simulink model "LCA_feature_mode"  (R2021a)
settings: Solver=VariableStepAuto  StartTime=0.0  StopTime=sim_time  RelTol=1e-3
values from neighbouring files (symbols this model uses):
  c_f = 155494.663    [LCA_init.m]    (also in MPC_init.m; week6_init.m)
  c_r = 1554494.663    [LCA_init.m]    (also in MPC_init.m; week6_init.m)
  I_z = 1436.24    [LCA_init.m]    (also in MPC_init.m; week6_init.m)
  L = 4.7    [LCA_init.m]    (also in LCA_lateral_movie_fcn.m = 5.7; PurePursuitModelInitialization.m; Pure_Pursiut_init.m; Stanley_control_init.m)
  l_f = 1.165    [LCA_init.m]    (also in MPC_init.m; week6_init.m)
  l_r = 1.165    [LCA_init.m]    (also in MPC_init.m; week6_init.m)
  ld = 15    [LCA_init.m]
  m = 1084    [Headway_Controller_Design.m]    (also in LCA_init.m = 1140; MPC_init.m = 1140; PID_Controller.m = 1; Reduced_order_model.m)
  md = get_curvature(Vx, yaw_rate_pose, tRef)    [LCA_init.m]
  Ts = 0.1    [LCA_init.m]    (also in MPC_init.m = 26; PurePursuitModelInitialization.m = 9; Pure_Pursiut_init.m = 9; Stanley_control_init.m = 1.6)
  Vx = 25    [LCA_init.m]    (also in MPC_init.m = 10; week6_init.m = 30)
  xRef = refPose(1,:)    [LCA_init.m]    (also in MPC_init.m; PurePursuitModelInitialization.m = refPose(:,1); Pure_Pursiut_init.m; Stanley_control_init.m = refpose(1,:))
  yRef = refPose(2,:) + 2    [LCA_init.m]    (also in MPC_init.m; PurePursuitModelInitialization.m = -refPose(:,2); Pure_Pursiut_init.m = refPose(2,:); Stanley_control_init.m = refpose(2,:))
undefined symbols (not defined in the file or in its folder): sigbuilder_block
libraries: simulink x2, mpcadaslib x1, robotalgslib x1, autolibshared x1
settings Model: Creator=User  LastModifiedBy=User

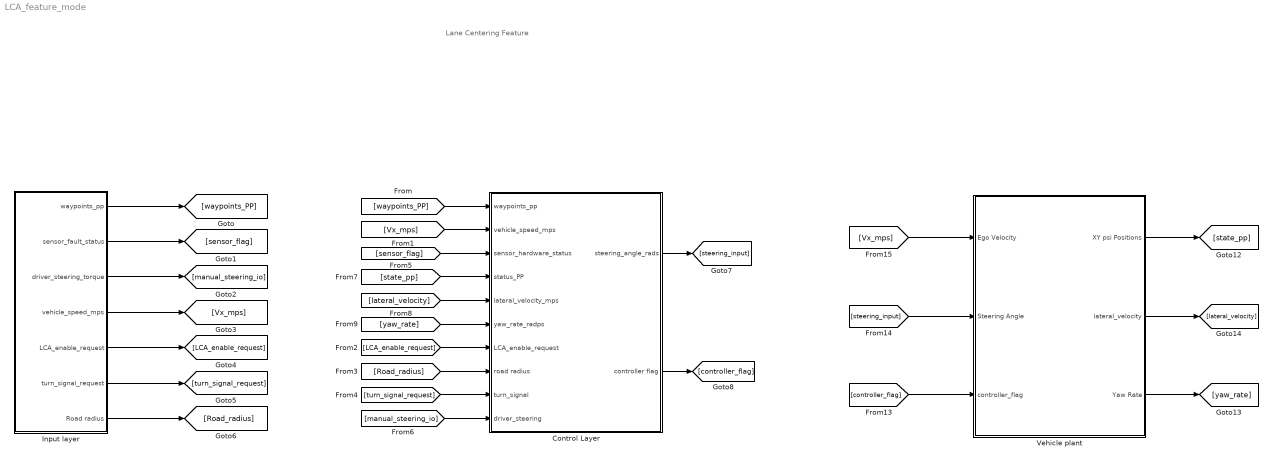
== system LCA_feature_mode ==
  note: Lane Centering Feature
  "\tControl Layer" : Subsystem
  Input layer : Subsystem
  Vehicle plant : Subsystem
  wires:
  Input layer/1(waypoints_pp) -> [waypoints_PP]
  Input layer/2(sensor_fault_status) -> [sensor_flag]
  Input layer/3(driver_steering_torque) -> [manual_steering_io]
  Input layer/4(vehicle_speed_mps) -> [Vx_mps]
  Input layer/5(LCA_enable_request) -> [LCA_enable_request]
  Input layer/6(turn_signal_request) -> [turn_signal_request]
  Input layer/7(Road radius) -> [Road_radius]
  [waypoints_PP] -> "\tControl Layer"/1(waypoints_pp)
  [Vx_mps] -> "\tControl Layer"/2(vehicle_speed_mps)
  [LCA_enable_request] -> "\tControl Layer"/7(LCA_enable_request)
  [Road_radius] -> "\tControl Layer"/8(road radius)
  [turn_signal_request] -> "\tControl Layer"/9(turn_signal)
  [sensor_flag] -> "\tControl Layer"/3(sensor_hardware_status)
  [manual_steering_io] -> "\tControl Layer"/10(driver_steering)
  [state_pp] -> "\tControl Layer"/4(status_PP)
  [lateral_velocity] -> "\tControl Layer"/5(lateral_velocity_mps)
  [yaw_rate] -> "\tControl Layer"/6(yaw_rate_radps)
  "\tControl Layer"/1(steering_angle_rads) -> [steering_input]
  "\tControl Layer"/2(controller flag) -> [controller_flag]
  Vehicle plant/1(XY psi Positions) -> [state_pp]
  Vehicle plant/3(Yaw Rate) -> [yaw_rate]
  [steering_input] -> Vehicle plant/2(Steering Angle)
  [Vx_mps] -> Vehicle plant/1(Ego Velocity)
  Vehicle plant/2(lateral_velocity) -> [lateral_velocity]
  [controller_flag] -> Vehicle plant/3(controller_flag)

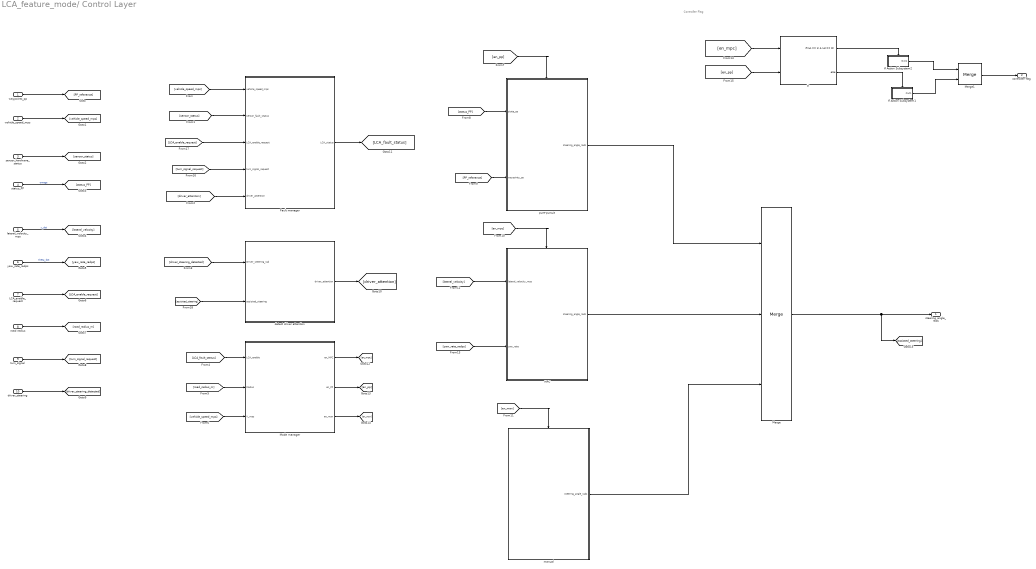
== system LCA_feature_mode/	Control Layer ==
  note: Controller Flag
  waypoints_pp : Inport
  vehicle_speed_mps : Inport  Port=2
  sensor_hardware_status : Inport  Port=3
  status_PP : Inport  Port=4
  lateral_velocity_mps : Inport  Port=5
  yaw_rate_radps : Inport  Port=6
  LCA_enable_request : Inport  Port=7
  road radius : Inport  Port=8
  turn_signal : Inport  Port=9
  driver_steering : Inport  Port=10
  Fault manager : Subsystem
  If : If  NumInputs=2  IfExpression=(u1 == 1) & (u2 == 0)
  If Action Subsystem1 : Subsystem  TreatAsAtomicUnit=on
  If Action Subsystem2 : Subsystem  TreatAsAtomicUnit=on
  MPC : Subsystem
  Merge : Merge  Inputs=3
  Merge1 : Merge
  Mode manager : Subsystem
  detect driver attention : Subsystem
  manual : Subsystem
  pure-pursuit : Subsystem
  steering_angle_rads : Outport
  controller flag : Outport  Port=2
  wires:
  waypoints_pp/1 -> [PP_reference]
  vehicle_speed_mps/1 -> [vehicle_speed_mps]
  sensor_hardware_status/1 -> [sensor_status]
  status_PP/1 -> [status_PP]  "omega"
  lateral_velocity_mps/1 -> [lateral_velocity]  "y_dot"
  yaw_rate_radps/1 -> [yaw_rate_radps]  "theta_dot"
  LCA_enable_request/1 -> [LCA_enable_request]
  road radius/1 -> [road_radius_m]
  turn_signal/1 -> [turn_signal_request]
  driver_steering/1 -> [driver_steering_detected]
  [vehicle_speed_mps] -> Fault manager/1(vehicle_speed_mps)
  [sensor_status] -> Fault manager/2(sensor_fault_status)
  detect driver attention/1(driver_attention) -> [driver_attention]
  [driver_attention] -> Fault manager/5("\tdriver_attention")
  [driver_steering_detected] -> detect driver attention/1(Driver_steering_rad)
  Fault manager/1(LCA_status) -> [LCA_fault_status]
  [LCA_fault_status] -> Mode manager/1(LCA_enable)
  [road_radius_m] -> Mode manager/2(Radius)
  [vehicle_speed_mps] -> Mode manager/3(V_mps)
  Mode manager/1(en_MPC) -> [en_mpc]
  Mode manager/2(en_PP) -> [en_pp]
  Mode manager/3(en_man) -> [en_man]
  [en_pp] -> pure-pursuit/Enable
  [status_PP] -> pure-pursuit/1(state_pp)
  [PP_reference] -> pure-pursuit/2(waypoints_pp)
  pure-pursuit/1(steering_angle_rads) -> Merge/1
  MPC/1(steering_angle_rads) -> Merge/2
  [en_mpc] -> MPC/Enable
  [en_man] -> manual/Enable
  manual/1(steering_angle_rads) -> Merge/3
  Merge/1 -> [assisted_steering], steering_angle_rads/1
  [lateral_velocity] -> MPC/1(lateral_velocity_mps)
  [yaw_rate_radps] -> MPC/2(yaw_rate)
  [en_mpc] -> If/1
  [en_pp] -> If/2
  If/1 -> If Action Subsystem2/Action
  If Action Subsystem2/1(Out1) -> Merge1/1
  Merge1/1 -> controller flag/1
  If/2 -> If Action Subsystem1/Action
  If Action Subsystem1/1(Out1) -> Merge1/2
  [turn_signal_request] -> Fault manager/4("\tturn_signal_request")
  [LCA_enable_request] -> Fault manager/3("\tLCA_enable_request")
  [assisted_steering] -> detect driver attention/2(assisted_steering)

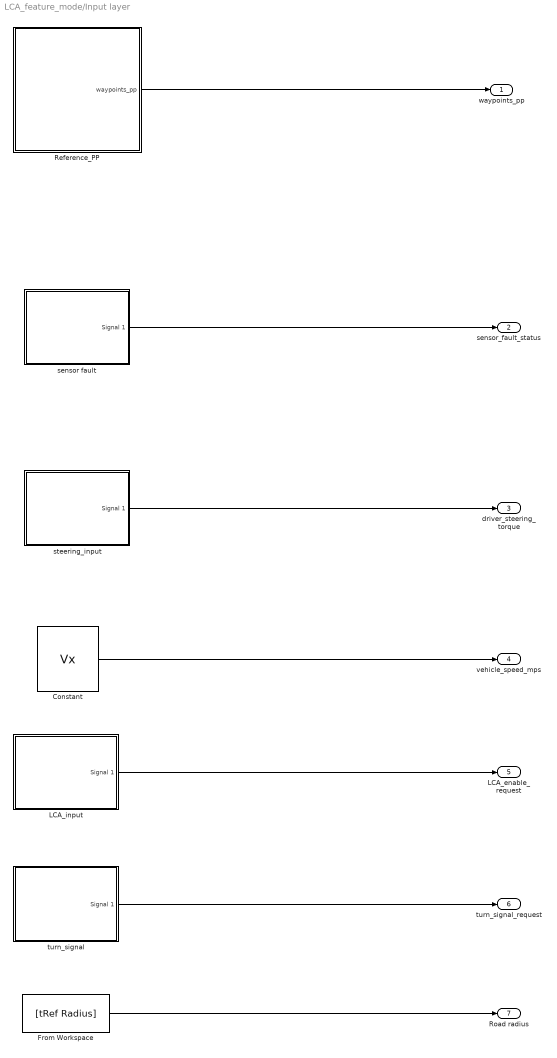
== system LCA_feature_mode/Input layer ==
  Constant : Constant  Value=Vx
  From Workspace : FromWorkspace  VariableName=[tRef Radius]  SampleTime=0.1
  LCA_input : Subsystem  Tag=STV Subsys  LoadFcn=sigbuilder_block('load');  StartFcn=sigbuilder_block('start');  StopFcn=sigbuilder_block('stop');  ClipboardFcn=sigbuilder_block('clipboard');  mask(Sigbuilder block){tuvar=[0:10]}
      mask help: Simulink:masks:SigbuilderBlock_MD
      mask init:
      | if ~strcmp(get_param(bdroot(gcbh),'SimulationStatus'),'stopped') tuvar = sigbuilder_block('maskInit'); end
      settings: CopyFcn=sigbuilder_block('copy');  DeleteFcn=sigbuilder_block('delete');  ModelCloseFcn=sigbuilder_block('modelClose');  PreSaveFcn=sigbuilder_block('preSave');  PauseFcn=sigbuilder_block('pause');  ContinueFcn=sigbuilder_block('continue');  NameChangeFcn=sigbuilder_block('namechange');  OpenFcn=sigbuilder_block('open',[309 216.75 550.5 359.25 ]);  CloseFcn=sigbuilder_block('close');
      mask Display: plot(0, 0, 100, 100,[2, 2, 32, 32, 2], [68, 8, 8, 68, 68],[32, 2], [38, 38], [32, 19, 2],[53, 60, 44], [32, 17, 17, 2],[16, 16, 31, 31]);txt = getActiveGroup(gcbh);text(2, 100, txt,'verticalAlignment', 'top');
  Reference_PP : Subsystem
  sensor fault : Subsystem  Tag=STV Subsys  LoadFcn=sigbuilder_block('load');  StartFcn=sigbuilder_block('start');  StopFcn=sigbuilder_block('stop');  ClipboardFcn=sigbuilder_block('clipboard');  mask(Sigbuilder block){tuvar=[0:10]}
      mask help: Simulink:masks:SigbuilderBlock_MD
      mask init:
      | if ~strcmp(get_param(bdroot(gcbh),'SimulationStatus'),'stopped') tuvar = sigbuilder_block('maskInit'); end
      settings: CopyFcn=sigbuilder_block('copy');  DeleteFcn=sigbuilder_block('delete');  ModelCloseFcn=sigbuilder_block('modelClose');  PreSaveFcn=sigbuilder_block('preSave');  PauseFcn=sigbuilder_block('pause');  ContinueFcn=sigbuilder_block('continue');  NameChangeFcn=sigbuilder_block('namechange');  OpenFcn=sigbuilder_block('open',[309 216.75 550.5 359.25 ]);  CloseFcn=sigbuilder_block('close');
      mask Display: plot(0, 0, 100, 100,[2, 2, 32, 32, 2], [68, 8, 8, 68, 68],[32, 2], [38, 38], [32, 19, 2],[53, 60, 44], [32, 17, 17, 2],[16, 16, 31, 31]);txt = getActiveGroup(gcbh);text(2, 100, txt,'verticalAlignment', 'top');
  steering_input : Subsystem  Tag=STV Subsys  LoadFcn=sigbuilder_block('load');  StartFcn=sigbuilder_block('start');  StopFcn=sigbuilder_block('stop');  ClipboardFcn=sigbuilder_block('clipboard');  mask(Sigbuilder block){tuvar=[0:10]}
      mask help: Simulink:masks:SigbuilderBlock_MD
      mask init:
      | if ~strcmp(get_param(bdroot(gcbh),'SimulationStatus'),'stopped') tuvar = sigbuilder_block('maskInit'); end
      settings: CopyFcn=sigbuilder_block('copy');  DeleteFcn=sigbuilder_block('delete');  ModelCloseFcn=sigbuilder_block('modelClose');  PreSaveFcn=sigbuilder_block('preSave');  PauseFcn=sigbuilder_block('pause');  ContinueFcn=sigbuilder_block('continue');  NameChangeFcn=sigbuilder_block('namechange');  OpenFcn=sigbuilder_block('open',[309 216.75 550.5 359.25 ]);  CloseFcn=sigbuilder_block('close');
      mask Display: plot(0, 0, 100, 100,[2, 2, 32, 32, 2], [68, 8, 8, 68, 68],[32, 2], [38, 38], [32, 19, 2],[53, 60, 44], [32, 17, 17, 2],[16, 16, 31, 31]);txt = getActiveGroup(gcbh);text(2, 100, txt,'verticalAlignment', 'top');
  turn_signal : Subsystem  Tag=STV Subsys  LoadFcn=sigbuilder_block('load');  StartFcn=sigbuilder_block('start');  StopFcn=sigbuilder_block('stop');  ClipboardFcn=sigbuilder_block('clipboard');  mask(Sigbuilder block){tuvar=[0:10]}
      mask help: Simulink:masks:SigbuilderBlock_MD
      mask init:
      | if ~strcmp(get_param(bdroot(gcbh),'SimulationStatus'),'stopped') tuvar = sigbuilder_block('maskInit'); end
      settings: CopyFcn=sigbuilder_block('copy');  DeleteFcn=sigbuilder_block('delete');  ModelCloseFcn=sigbuilder_block('modelClose');  PreSaveFcn=sigbuilder_block('preSave');  PauseFcn=sigbuilder_block('pause');  ContinueFcn=sigbuilder_block('continue');  NameChangeFcn=sigbuilder_block('namechange');  OpenFcn=sigbuilder_block('open',[309 216.75 550.5 359.25 ]);  CloseFcn=sigbuilder_block('close');
      mask Display: plot(0, 0, 100, 100,[2, 2, 32, 32, 2], [68, 8, 8, 68, 68],[32, 2], [38, 38], [32, 19, 2],[53, 60, 44], [32, 17, 17, 2],[16, 16, 31, 31]);txt = getActiveGroup(gcbh);text(2, 100, txt,'verticalAlignment', 'top');
  waypoints_pp : Outport
  sensor_fault_status : Outport  Port=2
  driver_steering_torque : Outport  Port=3
  vehicle_speed_mps : Outport  Port=4
  LCA_enable_request : Outport  Port=5
  turn_signal_request : Outport  Port=6
  Road radius : Outport  Port=7
  wires:
  Reference_PP/1(waypoints_pp) -> waypoints_pp/1
  sensor fault/1(Signal 1) -> sensor_fault_status/1
  steering_input/1(Signal 1) -> driver_steering_torque/1
  Constant/1 -> vehicle_speed_mps/1
  LCA_input/1(Signal 1) -> LCA_enable_request/1
  turn_signal/1(Signal 1) -> turn_signal_request/1
  From Workspace/1 -> Road radius/1

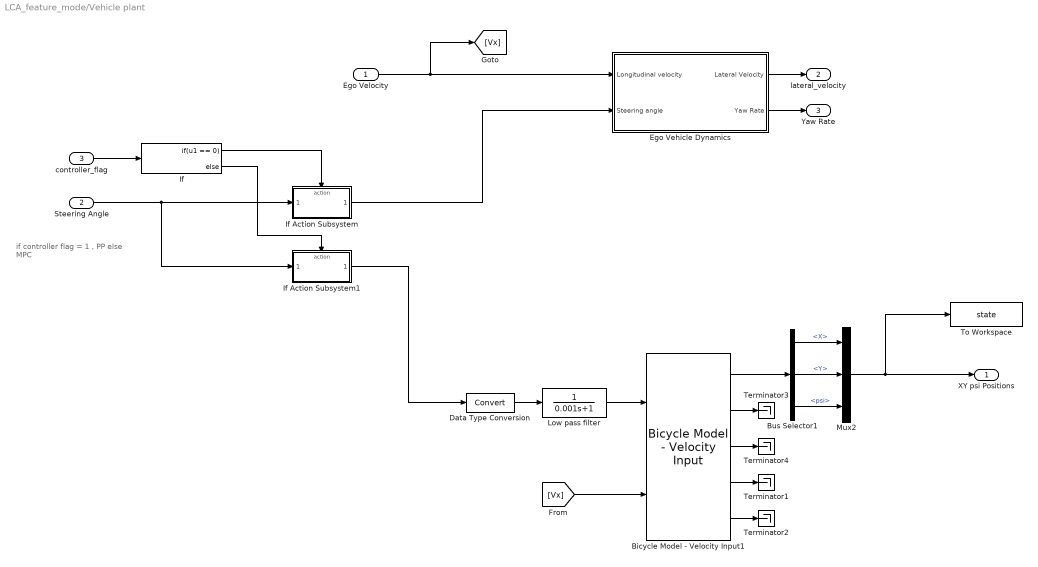
== system LCA_feature_mode/Vehicle plant ==
  note: if controller flag = 1 , PP
      | else MPC
  Ego Velocity : Inport
  Steering Angle : Inport  Port=2
  controller_flag : Inport  Port=3
  Bicycle Model - Velocity Input1 : autolibshared/Bicycle Model - Velocity Input  trackMode=Single (bicycle)  inputMode=External longitudinal forces  frontSteerMode=on  rearSteerMode=off  windMode=off  muMode=off  extFMode=off  extMMode=off  aMode=3  NF=2  NR=2  m=m  a=l_f  b=l_r  h=0.35  X_o=X_o  xdot_o=0  CalphaMode=off  sigmaMode=on  w=[1.4,1.4]  Cy_f=c_f  Cy_r=c_r  sigma_f=.1  sigma_r=.1  alpha_f_brk=[-.1 .1]  Cy_f_data=[-9e3 9e3]  alpha_r_brk=[-.1 .1]  Cy_r_data=[-9e3 9e3]  Y_o=Y_o  ydot_o=0  Izz=I_z  psi_o=0  r_o=0  Af=2  Cd=.3  Cl=.1  Cpm=.1  beta_w=[0:0.01:0.3]  Cs=[0:0.03:0.9]  Cym=[0:0.01:0.3]  Pabs=101325  Tair=273  g=9.81  mu=1  xdot_tol=.01  Fznom=5000  Fxtire_sat=1e6  Fytire_sat=1e6  longOff=0  latOff=0  vertOff=0
      settings: SourceProductBaseCode=PW,MT,UV,VE,VP
  Bus Selector1 : BusSelector  OutputSignals=InertFrm.FrntAxl.Disp.X,InertFrm.FrntAxl.Disp.Y,InertFrm.Cg.Ang.psi
  Data Type Conversion : DataTypeConversion
  Ego Vehicle Dynamics : Subsystem
  If : If  IfExpression=u1 == 0
  If Action Subsystem : Subsystem  TreatAsAtomicUnit=on
  If Action Subsystem1 : Subsystem  TreatAsAtomicUnit=on
  Low pass filter : TransferFcn  Denominator=[0.001 1]
  Mux2 : Mux  Inputs=3
  Terminator{1..4} (4 alike) : Terminator
  To Workspace : ToWorkspace  VariableName=state  SampleTime=-1
  XY psi Positions : Outport  Unit=m  VectorParamsAs1DForOutWhenUnconnected=off
  lateral_velocity : Outport  Port=2  Unit=m/s  VectorParamsAs1DForOutWhenUnconnected=off
  Yaw Rate : Outport  Port=3  Unit=degree/s  VectorParamsAs1DForOutWhenUnconnected=off
  wires:
  Bicycle Model - Velocity Input1/3 -> Terminator4/1
  Bicycle Model - Velocity Input1/2 -> Terminator3/1
  Data Type Conversion/1 -> Low pass filter/1
  Mux2/1 -> To Workspace/1, XY psi Positions/1
  Bicycle Model - Velocity Input1/1 -> Bus Selector1/1
  Low pass filter/1 -> Bicycle Model - Velocity Input1/1
  Bicycle Model - Velocity Input1/5 -> Terminator2/1
  Bus Selector1/1 -> Mux2/1  "<X>"
  Bus Selector1/2 -> Mux2/2  "<Y>"
  Bicycle Model - Velocity Input1/4 -> Terminator1/1
  Bus Selector1/3 -> Mux2/3  "<psi>"
  Ego Velocity/1 -> [Vx], Ego Vehicle Dynamics/1(Longitudinal velocity)
  Ego Vehicle Dynamics/2(Yaw Rate) -> Yaw Rate/1
  Ego Vehicle Dynamics/1(Lateral Velocity) -> lateral_velocity/1
  [Vx] -> Bicycle Model - Velocity Input1/2
  controller_flag/1 -> If/1
  Steering Angle/1 -> If Action Subsystem1/1(Steering Angle), If Action Subsystem/1(Steering Angle)
  If/1 -> If Action Subsystem/Action
  If/2 -> If Action Subsystem1/Action
  If Action Subsystem/1(steering angle to ego dynamics) -> Ego Vehicle Dynamics/2(Steering angle)
  If Action Subsystem1/1(wheenangle) -> Data Type Conversion/1

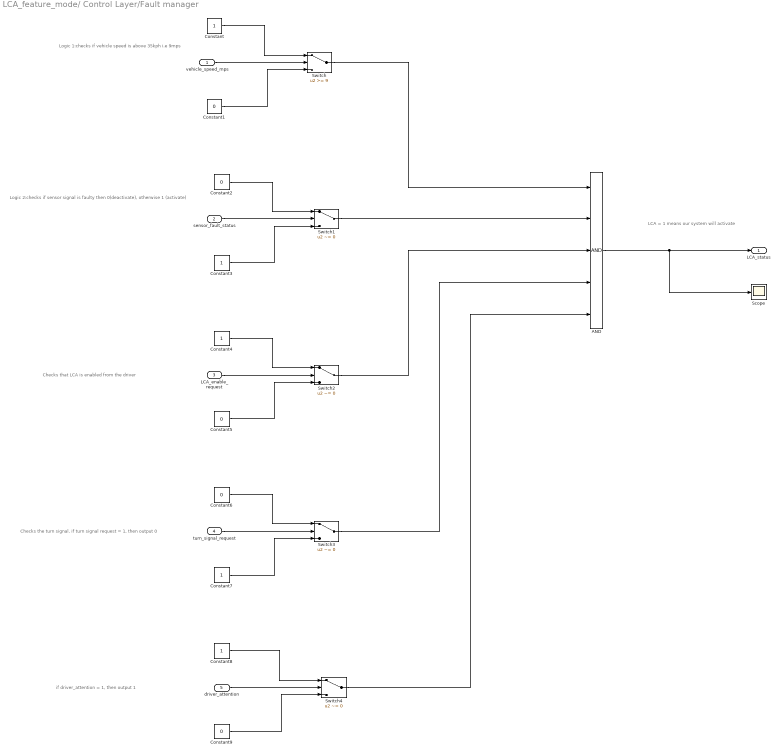
== system LCA_feature_mode/	Control Layer/Fault manager ==
  note: Logic 1:checks if vehicle speed is above 35kph i.e 9mps
  note: Logic 2:checks if sensor signal is faulty then 0(deactivate), otherwise 1 (activate)
  note: Checks that LCA is enabled from the driver
  note: Checks the turn signal. if turn signal request = 1, then output 0
  note: if driver_attention = 1, then output 1
  note: LCA = 1 means our system will activate
  vehicle_speed_mps : Inport
  sensor_fault_status : Inport  Port=2
  "\tLCA_enable_request" : Inport  Port=3
  "\tturn_signal_request" : Inport  Port=4
  "\tdriver_attention" : Inport  Port=5
  AND : Logic  Inputs=5  AllPortsSameDT=off  OutDataTypeStr=boolean
  Constant{,3..4,7..8} (5 alike) : Constant
  Constant{1..2,5..6,9} (5 alike) : Constant  Value=0
  Scope : Scope
  Switch : Switch  Threshold=9
  Switch{1..4} (4 alike) : Switch  Criteria=u2 ~= 0
  LCA_status : Outport
  wires:
  vehicle_speed_mps/1 -> Switch/2
  Constant/1 -> Switch/1
  Constant1/1 -> Switch/3
  Constant3/1 -> Switch1/3
  Constant2/1 -> Switch1/1
  sensor_fault_status/1 -> Switch1/2
  "\tLCA_enable_request"/1 -> Switch2/2
  Constant4/1 -> Switch2/1
  Constant5/1 -> Switch2/3
  Constant7/1 -> Switch3/3
  Constant6/1 -> Switch3/1
  "\tturn_signal_request"/1 -> Switch3/2
  "\tdriver_attention"/1 -> Switch4/2
  Constant8/1 -> Switch4/1
  Constant9/1 -> Switch4/3
  Switch/1 -> AND/1
  Switch1/1 -> AND/2
  Switch2/1 -> AND/3
  Switch3/1 -> AND/4
  Switch4/1 -> AND/5
  AND/1 -> Scope/1, LCA_status/1

== system LCA_feature_mode/	Control Layer/If Action Subsystem1 ==
  Action Port : ActionPort  ActionPortLabel=else
  Constant : Constant
  Out1 : Outport
  wires:
  Constant/1 -> Out1/1

== system LCA_feature_mode/	Control Layer/If Action Subsystem2 ==
  Action Port : ActionPort  ActionPortLabel=if((u1 == 1) & (u2 == 0))
  Constant : Constant
  Out1 : Outport
  wires:
  Constant/1 -> Out1/1

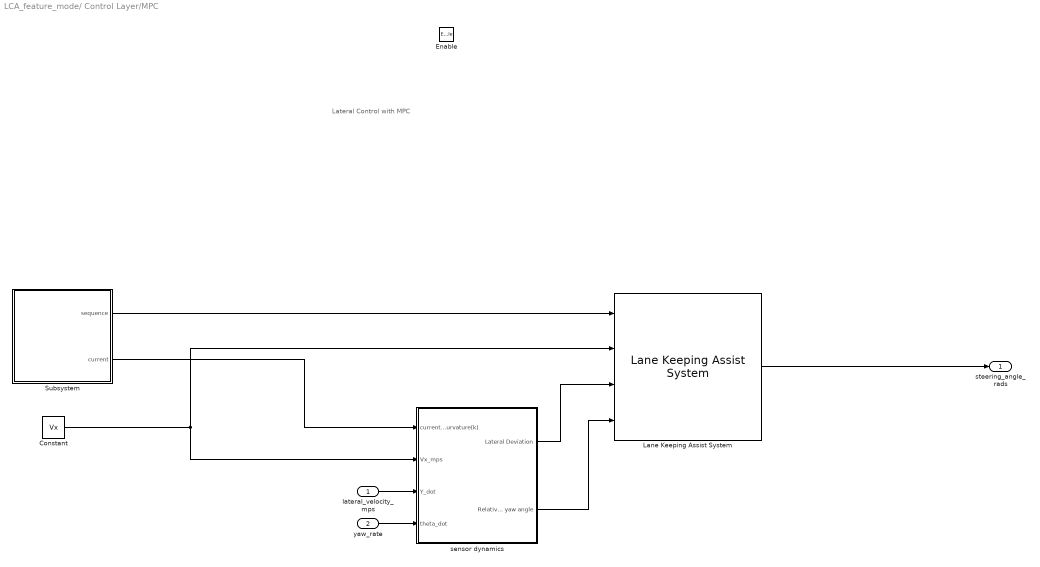
== system LCA_feature_mode/	Control Layer/MPC ==
  note: Lateral Control with MPC
  lateral_velocity_mps : Inport
  yaw_rate : Inport  Port=2
  Enable : EnablePort
  Constant : Constant  Value=Vx
  Lane Keeping Assist System : mpcadaslib/Lane Keeping Assist System  ModelType=Use vehicle parameters  VehicleMass=m  VehicleYawInertia=I_z  LengthToFront=l_f  LengthToRear=l_r  FrontTireStiffness=c_f  RearTireStiffness=c_r  EgoModelMatrixA=[-4.4021 ,-12.4603;1.3913,-5.1868]  EgoModelMatrixB=[24.1270;15.8609]  EgoModelMatrixC=[1,0;0,1]  InitialLongVel=Vx  TransportLag=0  MinSteering=-0.5  umin_ext=off  MaxSteering=0.5  umax_ext=off  Ts=0.1  PredictionHorizon=10  ControllerBehavior=0.500  suboptimal=off  maxiter=10  datatypeopt=double  optmode=off  trackmode=off
      settings: SourceProductBaseCode=MP
  Subsystem : Subsystem  mask{signal=md, ts=Ts, steps=10}
      mask prompts: signal "Signal name"; ts "Sampling time"; steps "Number of previewing steps"
      mask init:
      | ts = evalin('base',get_param(gcbh,'ts'));
      | signal = evalin('base',get_param(gcbh,'signal'));
      | steps = evalin('base',get_param(gcbh,'steps'));
      | data = mpc_previewer_maskinit(signal,ts);
      mask Display:
      | fprintf('Future\nsample\nextractor');
      | port_label('output', 1, 'seq')
      | port_label('output', 2, '@t')
  sensor dynamics : Subsystem
  steering_angle_rads : Outport
  wires:
  Lane Keeping Assist System/1 -> steering_angle_rads/1
  Constant/1 -> sensor dynamics/2(Vx_mps), Lane Keeping Assist System/2
  sensor dynamics/1(Lateral Deviation) -> Lane Keeping Assist System/3
  sensor dynamics/2(Relative yaw angle) -> Lane Keeping Assist System/4
  lateral_velocity_mps/1 -> sensor dynamics/3(Y_dot)
  yaw_rate/1 -> sensor dynamics/4(theta_dot)
  Subsystem/2(current) -> sensor dynamics/1(current_curvature(k))
  Subsystem/1(sequence) -> Lane Keeping Assist System/1

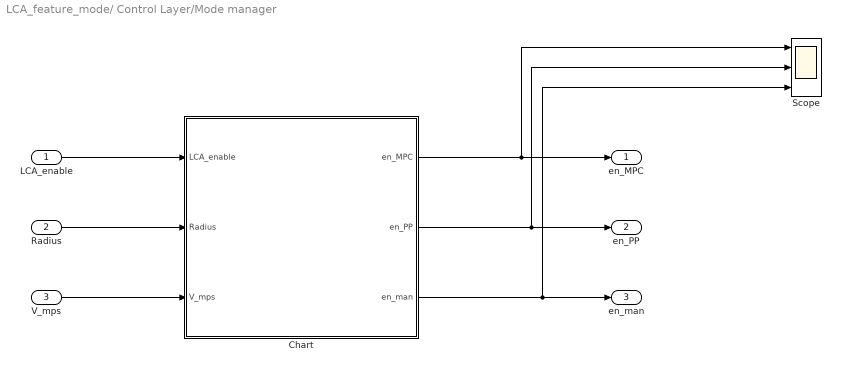
== system LCA_feature_mode/	Control Layer/Mode manager ==
  LCA_enable : Inport
  Radius : Inport  Port=2
  V_mps : Inport  Port=3
  Chart : Stateflow chart  TreatAsAtomicUnit=on
  Scope : Scope  NumInputPorts=3
  en_MPC : Outport
  en_PP : Outport  Port=2
  en_man : Outport  Port=3
  wires:
  LCA_enable/1 -> Chart/1(LCA_enable)
  Radius/1 -> Chart/2(Radius)
  V_mps/1 -> Chart/3(V_mps)
  Chart/1(en_MPC) -> Scope/1, en_MPC/1
  Chart/2(en_PP) -> Scope/2, en_PP/1
  Chart/3(en_man) -> Scope/3, en_man/1

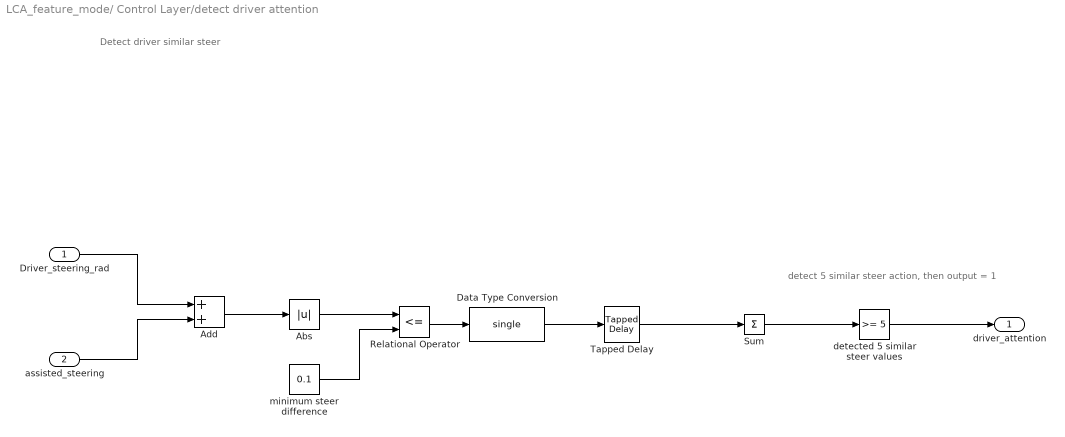
== system LCA_feature_mode/	Control Layer/detect driver attention ==
  note: detect 5 similar steer action, then output = 1
  note: Detect driver similar steer
  Driver_steering_rad : Inport
  assisted_steering : Inport  Port=2
  Abs : Abs
  Add : Sum
  Data Type Conversion : DataTypeConversion  OutDataTypeStr=single
  Relational Operator : RelationalOperator  Operator=<=  OutDataTypeStr=boolean  RndMeth=Simplest
  Sum : Sum  Inputs=+
  Tapped Delay : simulink/Discrete/Tapped Delay  vinit=0.0  samptime=-1  NumDelays=5  DelayOrder=Oldest  includeCurrent=off
  detected 5 similar steer values : simulink/Logic and Bit Operations/Compare To Constant  relop=>=  const=5  OutDataTypeStr=boolean
  minimum steer difference : Constant  Value=0.1
  driver_attention : Outport
  wires:
  Driver_steering_rad/1 -> Add/1
  assisted_steering/1 -> Add/2
  Add/1 -> Abs/1
  Abs/1 -> Relational Operator/1
  minimum steer difference/1 -> Relational Operator/2
  Relational Operator/1 -> Data Type Conversion/1
  Data Type Conversion/1 -> Tapped Delay/1
  Tapped Delay/1 -> Sum/1
  Sum/1 -> detected 5 similar steer values/1
  detected 5 similar steer values/1 -> driver_attention/1

== system LCA_feature_mode/	Control Layer/manual ==
  Enable : EnablePort
  Constant : Constant  Value=0
  steering_angle_rads : Outport
  wires:
  Constant/1 -> steering_angle_rads/1

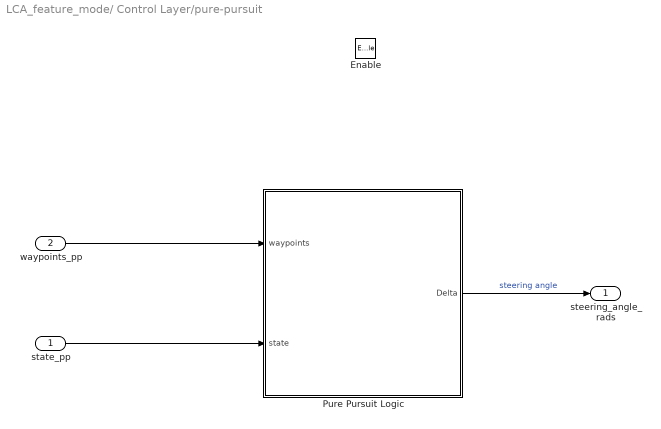
== system LCA_feature_mode/	Control Layer/pure-pursuit ==
  state_pp : Inport
  waypoints_pp : Inport  Port=2
  Enable : EnablePort
  Pure Pursuit Logic : Subsystem
  steering_angle_rads : Outport
  wires:
  state_pp/1 -> Pure Pursuit Logic/2(state)
  waypoints_pp/1 -> Pure Pursuit Logic/1(waypoints)
  Pure Pursuit Logic/1(Delta) -> steering_angle_rads/1  "steering angle"

== system LCA_feature_mode/Input layer/LCA_input ==
  Demux : Demux  Tag=STV Demux  Outputs=1
      settings: DisplayOption=none
  FromWs : FromWorkspace  Tag=STV FromWs  VariableName=tuvar
      SigBuilderData=|
      | common.afterFinalStr = 'Extrapolate'
      | common.sampleTime = 0
      | dataSet.timeRange = [0 10]
      | dataSet.name = 'Group 1'
      | sbobj.Groups.Name = 'Group 1'
      | sbobj.Groups.Signals.Name = 'Signal 1'
      | sbobj.Groups.Signals.XData = [0 4 4 6 6 10]
      | sbobj.Groups.Signals.YData = [0 0 1 1 0 0]
  Signal 1 : Outport  Tag=STV Outport
  wires:
  Demux/1 -> Signal 1/1
  FromWs/1 -> Demux/1

== system LCA_feature_mode/Input layer/Reference_PP ==
  Constant : Constant  Value=xRef  SampleTime=0.1
  Constant1 : Constant  Value=yRef  SampleTime=0.1
  Matrix Concatenate : Concatenate  Mode=Multidimensional array  ConcatenateDimension=2
  waypoints_pp : Outport
  wires:
  Constant/1 -> Matrix Concatenate/1
  Constant1/1 -> Matrix Concatenate/2
  Matrix Concatenate/1 -> waypoints_pp/1

== system LCA_feature_mode/Input layer/sensor fault ==
  Demux : Demux  Tag=STV Demux  Outputs=1
      settings: DisplayOption=none
  FromWs : FromWorkspace  Tag=STV FromWs  VariableName=tuvar
      SigBuilderData=|
      | common.afterFinalStr = 'Extrapolate'
      | common.sampleTime = 0
      | dataSet.timeRange = [0 10]
      | dataSet.name = 'Group 1'
      | sbobj.Groups.Name = 'Group 1'
      | sbobj.Groups.Signals.Name = 'Signal 1'
      | sbobj.Groups.Signals.XData = [0 4 4 6 6 10]
      | sbobj.Groups.Signals.YData = [0 0 1 1 0 0]
  Signal 1 : Outport  Tag=STV Outport
  wires:
  Demux/1 -> Signal 1/1
  FromWs/1 -> Demux/1

== system LCA_feature_mode/Input layer/steering_input ==
  Demux : Demux  Tag=STV Demux  Outputs=1
      settings: DisplayOption=none
  FromWs : FromWorkspace  Tag=STV FromWs  VariableName=tuvar
      SigBuilderData=|
      | common.afterFinalStr = 'Extrapolate'
      | common.sampleTime = 0
      | dataSet.timeRange = [0 10]
      | dataSet.name = 'Group 1'
      | sbobj.Groups.Name = 'Group 1'
      | sbobj.Groups.Signals.Name = 'Signal 1'
      | sbobj.Groups.Signals.XData = [0 4 4 6 6 10]
      | sbobj.Groups.Signals.YData = [0 0 1 1 0 0]
  Signal 1 : Outport  Tag=STV Outport
  wires:
  FromWs/1 -> Demux/1
  Demux/1 -> Signal 1/1

== system LCA_feature_mode/Input layer/turn_signal ==
  Demux : Demux  Tag=STV Demux  Outputs=1
      settings: DisplayOption=none
  FromWs : FromWorkspace  Tag=STV FromWs  VariableName=tuvar
      SigBuilderData=|
      | common.afterFinalStr = 'Extrapolate'
      | common.sampleTime = 0
      | dataSet.timeRange = [0 10]
      | dataSet.name = 'Group 1'
      | sbobj.Groups.Name = 'Group 1'
      | sbobj.Groups.Signals.Name = 'Signal 1'
      | sbobj.Groups.Signals.XData = [0 4 4 6 6 10]
      | sbobj.Groups.Signals.YData = [0 0 1 1 0 0]
  Signal 1 : Outport  Tag=STV Outport
  wires:
  FromWs/1 -> Demux/1
  Demux/1 -> Signal 1/1

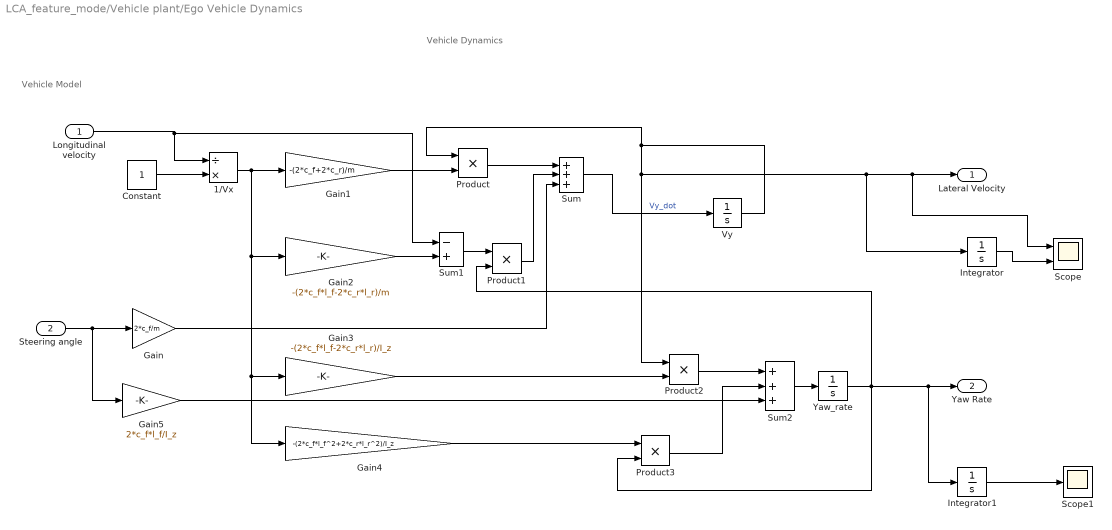
== system LCA_feature_mode/Vehicle plant/Ego Vehicle Dynamics ==
  note: Vehicle Model
  note: Vehicle Dynamics
  Longitudinal velocity : Inport
  Steering angle : Inport  Port=2
  1/Vx : Product  Inputs=/*
  Constant : Constant
  Gain : Gain  Gain=2*c_f/m
  Gain1 : Gain  Gain=-(2*c_f+2*c_r)/m
  Gain2 : Gain  Gain=-(2*c_f*l_f-2*c_r*l_r)/m
  Gain3 : Gain  Gain=-(2*c_f*l_f-2*c_r*l_r)/I_z
  Gain4 : Gain  Gain=-(2*c_f*l_f^2+2*c_r*l_r^2)/I_z
  Gain5 : Gain  Gain=2*c_f*l_f/I_z
  Integrator : Integrator
  Integrator1 : Integrator
  Product{,1..3} (4 alike) : Product
  Scope : Scope  NumInputPorts=2
  Scope1 : Scope
  Sum : Sum  Inputs=+++
  Sum1 : Sum  Inputs=-+
  Sum2 : Sum  Inputs=+++
  Vy : Integrator
  "Yaw_rate " : Integrator
  Lateral Velocity : Outport  VectorParamsAs1DForOutWhenUnconnected=off
  Yaw Rate : Outport  Port=2  VectorParamsAs1DForOutWhenUnconnected=off
  wires:
  Sum2/1 -> "Yaw_rate "/1
  Gain2/1 -> Sum1/2
  Gain4/1 -> Product3/1
  Constant/1 -> 1/Vx/2
  Gain3/1 -> Product2/2
  1/Vx/1 -> Gain4/1, Gain3/1, Gain2/1, Gain1/1
  Product2/1 -> Sum2/1
  Product3/1 -> Sum2/2
  Gain5/1 -> Sum2/3
  Sum1/1 -> Product1/1
  "Yaw_rate "/1 -> Product3/2, Integrator1/1, Yaw Rate/1, Product1/2
  Gain/1 -> Sum/3
  Steering angle/1 -> Gain/1, Gain5/1
  Gain1/1 -> Product/2
  Product/1 -> Sum/1
  Vy/1 -> Product/1, Integrator/1, Scope/1, Lateral Velocity/1, Product2/1
  Sum/1 -> Vy/1  "Vy_dot"
  Longitudinal velocity/1 -> Sum1/1, 1/Vx/1
  Product1/1 -> Sum/2
  Integrator/1 -> Scope/2
  Integrator1/1 -> Scope1/1

== system LCA_feature_mode/Vehicle plant/If Action Subsystem ==
  note: for MPC feedback
  Steering Angle : Inport
  Action Port : ActionPort  ActionPortLabel=if(u1 == 0)
  steering angle to ego dynamics : Outport
  wires:
  Steering Angle/1 -> steering angle to ego dynamics/1

== system LCA_feature_mode/Vehicle plant/If Action Subsystem1 ==
  note: for the PP feedback to vehicle dynamics block
  Steering Angle : Inport
  Action Port : ActionPort  ActionPortLabel=else
  wheenangle : Outport
  wires:
  Steering Angle/1 -> wheenangle/1

== system LCA_feature_mode/	Control Layer/MPC/Subsystem ==
  MATLAB Function : MATLAB Function  TreatAsAtomicUnit=on
  Memory1 : Memory  InheritSampleTime=on  LinearizeAsDelay=on
  sequence : Outport  VectorParamsAs1DForOutWhenUnconnected=off
  current : Outport  Port=2  VectorParamsAs1DForOutWhenUnconnected=off
  wires:
  MATLAB Function/2(first) -> current/1
  MATLAB Function/3(next_t) -> Memory1/1
  MATLAB Function/1(seq) -> sequence/1
  Memory1/1 -> MATLAB Function/1(t)

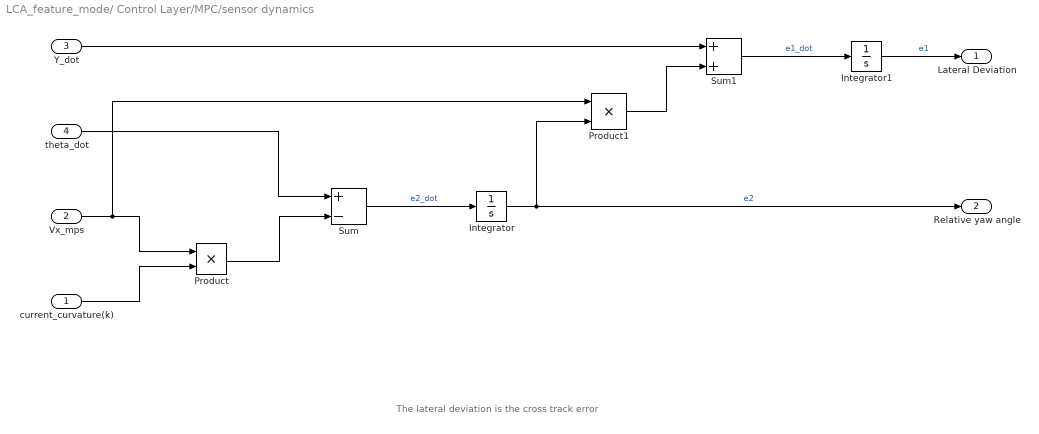
== system LCA_feature_mode/	Control Layer/MPC/sensor dynamics ==
  note: The lateral deviation is the cross track error
  current_curvature(k) : Inport
  Vx_mps : Inport  Port=2
  Y_dot : Inport  Port=3
  theta_dot : Inport  Port=4
  Integrator : Integrator
  Integrator1 : Integrator
  Product : Product
  Product1 : Product
  Sum : Sum  Inputs=+-
  Sum1 : Sum
  Lateral Deviation : Outport
  Relative yaw angle : Outport  Port=2
  wires:
  Vx_mps/1 -> Product1/1, Product/1
  current_curvature(k)/1 -> Product/2
  Product/1 -> Sum/2
  theta_dot/1 -> Sum/1
  Sum/1 -> Integrator/1  "e2_dot"
  Integrator/1 -> Relative yaw angle/1, Product1/2  "e2"
  Y_dot/1 -> Sum1/1
  Product1/1 -> Sum1/2
  Sum1/1 -> Integrator1/1  "e1_dot"
  Integrator1/1 -> Lateral Deviation/1  "e1"

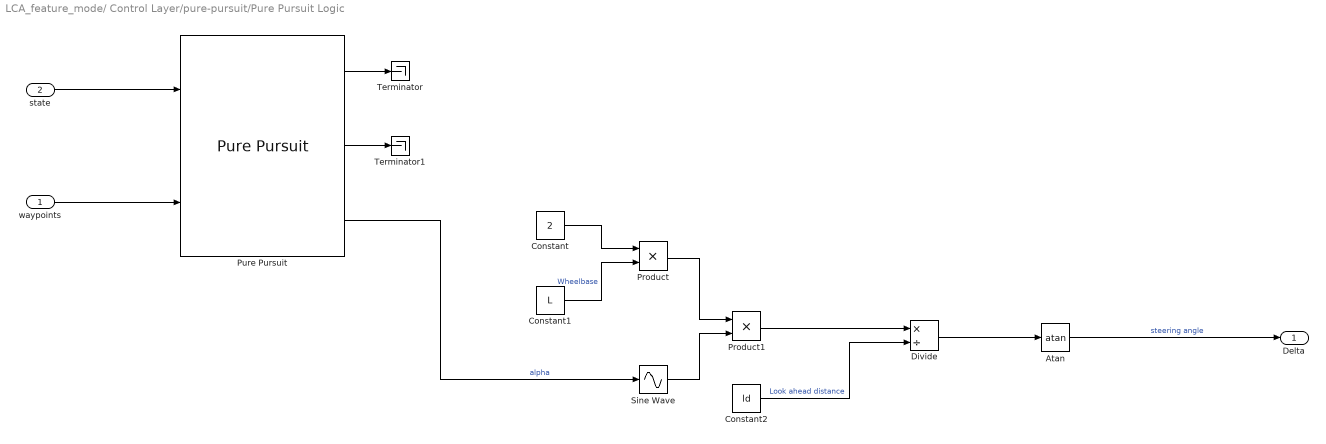
== system LCA_feature_mode/	Control Layer/pure-pursuit/Pure Pursuit Logic ==
  waypoints : Inport
  state : Inport  Port=2
  Atan : Trigonometry  Operator=atan
  Constant : Constant  Value=2
  Constant1 : Constant  Value=L
  Constant2 : Constant  Value=ld
  Divide : Product  Inputs=*/
  Product : Product
  Product1 : Product
  Pure Pursuit : robotalgslib/Pure Pursuit  DesiredLinearVelocity=Vx  MaxAngularVelocity=1.0  LookaheadDistance=ld  TargetDirPort=on  SimulateUsing=Code generation
  Sine Wave : Sin  TimeSource=Use external signal  SampleTime=0
  Terminator : Terminator
  Terminator1 : Terminator
  Delta : Outport
  wires:
  Atan/1 -> Delta/1  "steering angle"
  Divide/1 -> Atan/1
  Constant2/1 -> Divide/2  "Look ahead distance"
  Product1/1 -> Divide/1
  Sine Wave/1 -> Product1/2
  Product/1 -> Product1/1
  Constant1/1 -> Product/2  "Wheelbase"
  Constant/1 -> Product/1
  Pure Pursuit/3 -> Sine Wave/1  "alpha"
  Pure Pursuit/2 -> Terminator1/1
  Pure Pursuit/1 -> Terminator/1
  waypoints/1 -> Pure Pursuit/2
  state/1 -> Pure Pursuit/1

== matlab function LCA_feature_mode/	Control Layer/MPC/Subsystem/MATLAB Function ==
  settings: updateMethod=DISCRETE  sampleTime=ts
  data: data parameter; seq output; steps parameter; t input; first output; next_t output
function [seq,first,next_t] = fcn(data,steps,t)
%#codegen
[seq,first,next_t] = mpcblock_preview('md',data,steps,t);

== stateflow chart LCA_feature_mode/	Control Layer/Mode manager/Chart ==
  state LCA_off
    entry:en_man = true;
    en_PP = false;
    en_MPC = false;
  state LCA_On
    state PP
      entry:en_man = false;
      en_PP = true;
      en_MPC = false;
    state MPC
      entry:en_man = false;
      en_PP = false;
      en_MPC = true;
    (default) -> PP
    PP -> MPC : [((V_mps > 10) &&(Radius >= 1000)) || ((V_mps > 10) &&(Radius < 1000))]
    MPC -> PP : [((V_mps <= 10) &&(Radius >= 1000)) || ((V_mps <= 10) &&(Radius < 1000)) ]
  (default) -> LCA_off
  LCA_off -> LCA_On : [(LCA_enable) == 1]
  LCA_On -> LCA_off : [(LCA_enable) == 0]
  data: LCA_enable input; Radius input; V_mps input; en_MPC output; en_PP output; en_man output
